simulink model "simulation"  (R2023a)
settings: Solver=ode45  StartTime=0.0  StopTime=2  RelTol=1e-3
values from neighbouring files (symbols this model uses):
  K = -place(A, B, V)    [main.m]
  x0 = [0 ; pi/5 ; 0 ; 0]    [main.m]
undefined symbols (not defined in the file or in its folder): DiscIntNeverNeededParam
libraries: simulink x1
settings Model: Creator=ave9761  LastModifiedBy=ave9761

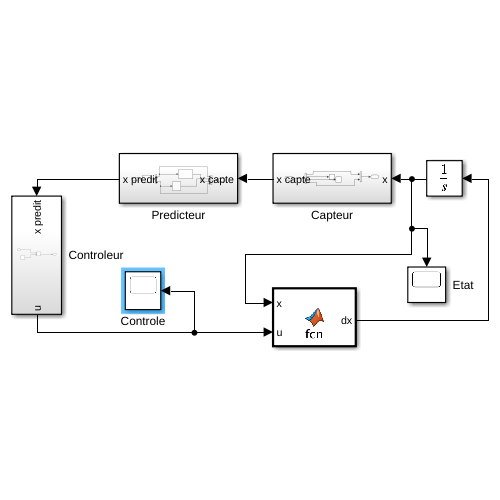
[thumbnail: Simulink's stored preview of the top-level diagram]
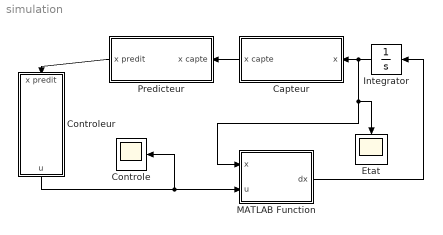
== system simulation ==
  Capteur : Subsystem
  Controle : Scope
  Controleur : Subsystem
  Etat : Scope
  Integrator : Integrator  InitialCondition=x0
  MATLAB Function : MATLAB Function  TreatAsAtomicUnit=on
  Predicteur : Subsystem
  wires:
  MATLAB Function/1(dx) -> Integrator/1
  Controleur/1(u) -> Controle/1, MATLAB Function/2(u)
  Capteur/1(x capte) -> Predicteur/1(x capte)
  Integrator/1 -> Etat/1, MATLAB Function/1(x), Capteur/1(x)
  Predicteur/1(x predit) -> Controleur/1(x predit)

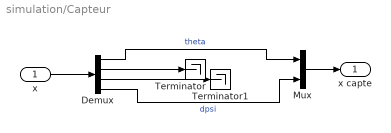
== system simulation/Capteur ==
  x : Inport
  Demux : Demux
  Mux : Mux  Inputs=2
  Terminator : Terminator
  Terminator1 : Terminator
  x capte : Outport
  wires:
  x/1 -> Demux/1
  Demux/2 -> Terminator/1
  Demux/3 -> Terminator1/1
  Demux/1 -> Mux/1  "theta"
  Demux/4 -> Mux/2  "dpsi"
  Mux/1 -> x capte/1

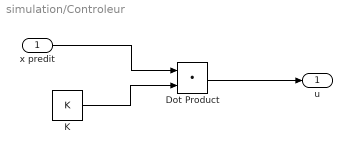
== system simulation/Controleur ==
  x predit : Inport
  Dot Product : DotProduct  OutDataTypeStr=Inherit: Inherit via internal rule
  K : Constant  Value=K
  u : Outport
  wires:
  x predit/1 -> Dot Product/1
  K/1 -> Dot Product/2
  Dot Product/1 -> u/1

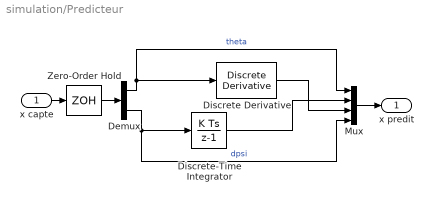
== system simulation/Predicteur ==
  x capte : Inport
  Demux : Demux  Outputs=2
  Discrete Derivative : simulink/Discrete/Discrete Derivative  gainval=1.0  ICPrevScaledInput=0.0  OutMin=[]  OutMax=[]  OutDataType=fixdt(1, 16)  OutScaling=2^-10  DoSatur=off
  Discrete-Time Integrator : DiscreteIntegrator  InitialCondition=x0(3)  SampleTime=-1  ICPrevOutput=DiscIntNeverNeededParam  ICPrevScaledInput=DiscIntNeverNeededParam
  Mux : Mux
  Zero-Order Hold : ZeroOrderHold  SampleTime=0.01
  x predit : Outport
  wires:
  Mux/1 -> x predit/1
  Demux/1 -> Discrete Derivative/1, Mux/1  "theta"
  Demux/2 -> Discrete-Time Integrator/1, Mux/4  "dpsi"
  x capte/1 -> Zero-Order Hold/1
  Zero-Order Hold/1 -> Demux/1
  Discrete Derivative/1 -> Mux/3
  Discrete-Time Integrator/1 -> Mux/2

== matlab function simulation/MATLAB Function ==
  data: x input; u input; dx output
function dx = fcn(x, u)

dx = fonction(x, u);
